simulink model "Controllers_Complete_Comparisons"  (R2021a)
settings: Solver=FixedStepAuto  StartTime=0  StopTime=1  FixedStep=0.002  RelTol=1e-3  EnableMultiTasking=on
PostLoadFcn:
  | qc_set_target_type(getConfigSet(bdroot, 'QUARC Default Target Configuration'));
values from neighbouring files (symbols this model uses):
  L_KF = KalmanFilter(sysest_ct, Q_KF, R_KF)    [LQR_comparison.m]    (also in main.m = Arco_KalmanFilter(sysest_ct, Q_KF, R_KF))
  L_obs = StateObserver(sysest_ct,obs_poles)    [LQR_comparison.m]    (also in main.m = StateObserver_JC(sysest_ct,obs_poles))
  Q_KF = eye(4)*10e-5    [LQR_comparison.m]    (also in main.m = eye(4))
  R_KF = eye(1)*10e-8    [LQR_comparison.m]    (also in main.m = eye(1))
  sysest = load("sysest09c_trick.mat").sysest    [LQR_comparison.m]    (also in main.m)
  sysest_ct = d2c(sysest)    [LQR_comparison.m]    (also in main.m)
  v_a_max = 13    [LQR_comparison.m]    (also in main.m = 15)
undefined symbols (not defined in the file or in its folder): DiscIntNeverNeededParam, HIL, k2, K_lqr, K_lqr_eta, K_lqr_eta_1, K_lqr_eta_2, K_lqr_eta_3, K_lqr_eta_4, K_lqr_x, K_lqr_x_1, K_lqr_x_2, K_lqr_x_3, K_lqr_x_4, K_lqrFF_eta, K_lqrFF_x, K_p, K_pp, K_pp_en_eta, K_pp_en_x, Kr2, L22, qc_get_step_size, sigbuilder_block
libraries: simulink_extras x15, quarc_library x4, cstblocks x1
settings Model: SimulationMode=external  ExtModeTrigDuration=5000  Creator=CFulford  LastModifiedBy=Andrea
settings SolverCC: AlgebraicLoopSolver=TrustRegion  PositivePriorityOrder=on
settings DataIOCC: LimitDataPoints=on  SaveFormat=Array  SignalLoggingSaveFormat=ModelDataLogs  ReturnWorkspaceOutputs=off
settings OptimizationCC: ExpressionDepthLimit=2147483647  InitFltsAndDblsToZero=on  LifeSpan=inf
settings DebuggingCC: SaveWithParameterizedLinksMsg=none  UnderspecifiedInitializationDetection=Classic  MergeDetectMultiDrivingBlocksExec=none  SolverPrmCheckMsg=warning  MultiTaskDSMMsg=warning  MultiTaskCondExecSysMsg=none  FcnCallInpInsideContextMsg=warning  StateNameClashWarn=warning  SFUnexpectedBacktrackingDiag=warning  SFNoUnconditionalDefaultTransitionDiag=warning  SFExecutionAtInitializationDiag=none  SFMachineParentedDataDiag=warning  ArithmeticOperatorsInVariantConditions=warning
settings HardwareCC: ProdBitPerPointer=32  ProdBitPerSizeT=32  ProdBitPerPtrDiffT=32  ProdLargestAtomicFloat=None  ProdIntDivRoundTo=Undefined  ProdEndianess=Unspecified  ProdWordSize=32  ProdHWDeviceType=32-bit Generic
settings ModelReferenceCC: PropagateSignalLabelsOutOfModel=off
settings SFSimCC: SimUseLocalCustomCode=off  CustomCodeUndefinedFunction=UseInterfaceOnly
settings RTWCC: Description=QUARC Win64 Target  SystemTargetFile=quarc_win64.tlc  TemplateMakefile=quarc_default_tmf  RTWUseLocalCustomCode=off
settings CodeAppCC: StateflowObjectComments=on
settings STFCustomTargetCC: TargetPreCompLibLocation=C:\PROGRA~3\QUARC\lib\2019b\win64\release  ConcurrentExecutionCompliant=on  CombineOutputUpdateFcns=on  CPPClassGenCompliant=on  GRTInterface=off  UseToolchainInfoCompliant=off  SystemTargetFile=quarc_win64.tlc
settings GRTTargetCC: TargetPreCompLibLocation=C:\PROGRA~3\QUARC\lib\2019b\win64\release  TargetLangStandard=C89/C90 (ANSI)  ParMdlRefBuildCompliant=off  CompOptLevelCompliant=off  MatFileLogging=off  UseToolchainInfoCompliant=off  ExtMode=on  ExtModeMexFile=quarc_comm
settings ConfigComp: CovMetricSettings=dw  CovSaveCumulativeToWorkspaceVar=on  CovSaveSingleToWorkspaceVar=on  CovExternalEMLEnable=off  CovSFcnEnable=off

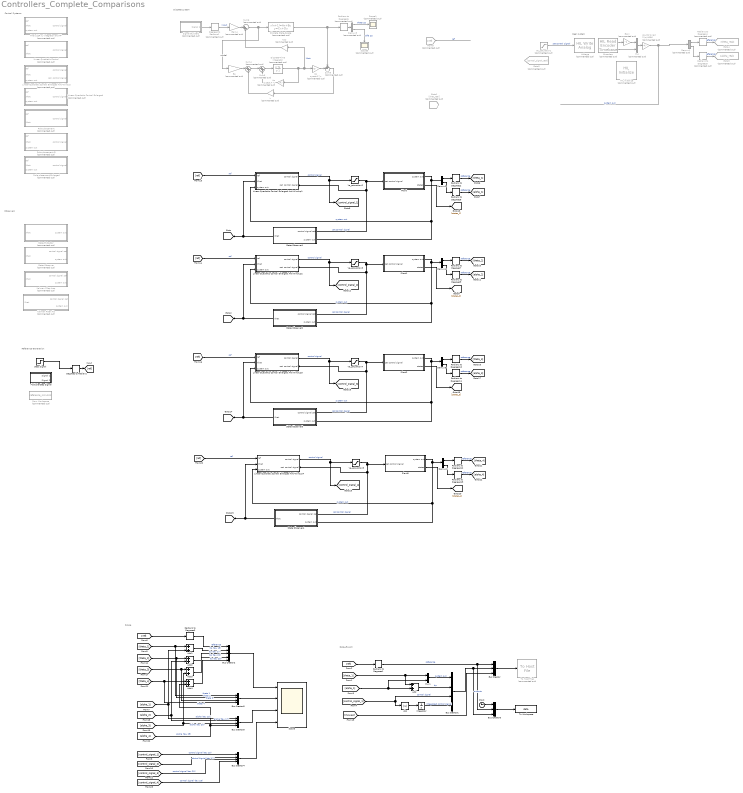
== system Controllers_Complete_Comparisons ==
  note: Real system
  note: Reference Generation
  note: Scope
  note: Control Systems
  note: Observers
  note: Discrete system
  note: model
  note: Data_Export
  Abs : Abs
  Add{,1..4} (5 alike) : Sum
  Ao : Gain  Commented=on  Gain=sysest.A  Multiplication=Matrix(K*u)
  Bo : Gain  Commented=on  Gain=sysest.B  Multiplication=Matrix(K*u)
  Bus Creator : BusCreator  Inputs=3
  Bus Creator{1,3..5} (4 alike) : BusCreator  Inputs=4
  Bus Creator2 : BusCreator  Inputs=5
  Bus Creator6 : BusCreator  Inputs=3
  Clock : Clock
  Co : Gain  Commented=on  Gain=sysest.C  Multiplication=Matrix(K*u)
  Degrees to Radians : simulink_extras/Transformations/Degrees to Radians
  Degrees to Radians1 : simulink_extras/Transformations/Degrees to Radians  Commented=on
  Demux1 : Demux  Commented=on  Outputs=2
  Demux{2,4..6} (4 alike) : Demux  Outputs=2
  Demux3 : Demux  Commented=on  Outputs=2
  Discrete State-Space : DiscreteStateSpace  Commented=on  A=sysest.A  B=sysest.B  C=sysest.C  D=sysest.D  SampleTime=0.002
  Discrete-Time Integrator : DiscreteIntegrator  Commented=on  SampleTime=0.002  ICPrevOutput=DiscIntNeverNeededParam  ICPrevScaledInput=DiscIntNeverNeededParam
  Encoders : quarc_library/Data Acquisition/Generic/Timebases/HIL Read Encoder Timebase  Commented=on  object_name=HIL-1  clock=0  channels=[0:1]  samples_in_buffer=max(ceil(1/qc_get_step_size), 1)  active=on  vector_output=off  data_type_mode=Inherit via back propagation  data_type=double
  Fire's LQR w/ integrator and FF : Subsystem  Commented=on
  From Workspace : FromWorkspace  Commented=on  VariableName=reference_simulink
  From9 : From  Commented=on  GotoTag=ref
  Gain : Gain  Commented=on  Gain=-1
  Gain4 : Gain  Commented=on  Gain=Kr2(1)
  Goto1 : Goto  Commented=on  GotoTag=Xhat_real
  Goto3 : Goto  Commented=on  GotoTag=alpha_real
  Goto4 : Goto  Commented=on  GotoTag=theta_real
  Goto5 : Goto  Commented=on  GotoTag=control_signal_real
  HIL Initialize : quarc_library/Data Acquisition/Generic/Configuration/HIL Initialize  Priority=-99  Commented=on  object_name=HIL-1  board_type=q2_usb  board_number=0  board_options=d0=digital;d1=digital;led=auto;update_rate=normal;decimation=1  exclusive=off  active=off  hardware_clocks=[0]  clock_modes=[]  initial_clock_frequencies=[]  set_clock_params_at_start=off  set_clock_params_at_switch_in=off  set_clock_frequencies_at_start=off  set_clock_frequencies_at_switch_in=off  analog_input_channels=[0:1]  analog_input_configurations=[]  analog_input_maximums=10  analog_input_minimums=-10  set_analog_input_params_at_start=on  set_analog_input_params_at_switch_in=off  analog_output_channels=[0:1]  analog_output_maximums=10  analog_output_minimums=-10  initial_analog_outputs=[0]  final_analog_outputs=[0]  watchdog_analog_outputs=0  set_analog_output_params_at_start=on  set_analog_output_params_at_switch_in=off  set_analog_outputs_at_start=on  set_analog_outputs_at_switch_in=off  set_analog_outputs_at_terminate=on  set_analog_outputs_at_switch_out=off  set_analog_outputs_on_watchdog=off  digital_input_channels=[]  digital_output_channels=[]  digital_output_configuration=[]  initial_digital_outputs=[1]  final_digital_outputs=[1]  watchdog_digital_outputs=[1]  set_digital_output_params_at_start=off  set_digital_output_params_at_switch_in=off  set_digital_outputs_at_start=on  set_digital_outputs_at_switch_in=off  set_digital_outputs_at_terminate=on  set_digital_outputs_at_switch_out=off  set_digital_outputs_on_watchdog=off  encoder_channels=[0:1]  quadrature=[4]  encoder_filter_frequency=[]  initial_encoder_counts=[0]  set_encoder_params_at_start=on  set_encoder_params_at_switch_in=off  set_encoder_counts_at_start=on  set_encoder_counts_at_switch_in=off  pwm_channels=[]  pwm_modes=[0]  pwm_frequency=1/0.020  pwm_configuration=[]  pwm_alignment=[]  pwm_polarity=[]  pwm_leading_deadband=[]  pwm_trailing_deadband=[]  initial_pwm_outputs=[0]  final_pwm_outputs=[0]  watchdog_pwm_outputs=[0]  set_pwm_params_at_start=on  set_pwm_params_at_switch_in=off  set_pwm_outputs_at_start=on  set_pwm_outputs_at_switch_in=off  set_pwm_outputs_at_terminate=on  set_pwm_outputs_at_switch_out=off  set_pwm_outputs_on_watchdog=off  other_output_channels=[]  initial_other_outputs=[]  final_other_outputs=[]  watchdog_other_outputs=[]  set_other_outputs_at_start=off  set_other_outputs_at_switch_in=off  set_other_outputs_at_terminate=off  set_other_outputs_at_switch_out=off  set_other_outputs_on_watchdog=off
  Integrator : Integrator
  Kalman Filter Alp : Subsystem  Commented=on
  Kalman Filter Arco : Subsystem  Commented=on
  Kpp : Gain  Commented=on  Gain=k2  Multiplication=Matrix(K*u)
  L : Gain  Commented=on  Gain=L22  Multiplication=Matrix(K*u)
  Linear Quadratic Control : Subsystem  Commented=on
  Linear Quadratic Control Enlarged : Subsystem  Commented=on
  Linear Quadratic Control Enlarged Anti-Windup : Subsystem  Commented=on
      settings: PortSchema="{\"entries\":[{\"content\":{\"sides\":[{\"content\":{\"connectorIds\":[\"In1\",\"In2\",\"In3\"]},\"type\":\"ConnectorPlacement.EquallySpacedRectSide\",\"uuid\":\"15b51522-458a-4f7c-a290-9c80724aecba\"},{\"content\":{\"connectorIds\":[\"Out1\",\"In4\"],\"side\":\"RIGHT\"},\"type\":\"ConnectorPlacement.EquallySpacedRectSide\",\"uuid\":\"ee497df3-c1d4-4daa-9165-c0ca341e658c\"},{\"content\":{\"connectorIds\":[],\"side\":\"TOP\"},\"type\":\"ConnectorPlacement.EquallySpacedRectSide\",\"uuid\":\"946f2086-2c09-46d1-b933-0f6497ae0c76\"}]},\"type\":\"ConnectorPlacement.EquallySpacedConnector\",\"uuid\":\"4633a66e-f116-47af-8162-46d62cad4c11\"}],\"packageUris\":[\"http://schema.mathworks.com/mf0/Connector/R2020b\"],\"version\":\"1.0\"}"
  Linear Quadratic Control Enlarged Anti-Windup1 : Subsystem
      settings: PortSchema="{\"entries\":[{\"content\":{\"sides\":[{\"content\":{\"connectorIds\":[\"In1\",\"In2\",\"In3\"]},\"type\":\"ConnectorPlacement.EquallySpacedRectSide\",\"uuid\":\"15b51522-458a-4f7c-a290-9c80724aecba\"},{\"content\":{\"connectorIds\":[\"Out1\",\"In4\"],\"side\":\"RIGHT\"},\"type\":\"ConnectorPlacement.EquallySpacedRectSide\",\"uuid\":\"ee497df3-c1d4-4daa-9165-c0ca341e658c\"},{\"content\":{\"connectorIds\":[],\"side\":\"TOP\"},\"type\":\"ConnectorPlacement.EquallySpacedRectSide\",\"uuid\":\"946f2086-2c09-46d1-b933-0f6497ae0c76\"}]},\"type\":\"ConnectorPlacement.EquallySpacedConnector\",\"uuid\":\"4633a66e-f116-47af-8162-46d62cad4c11\"}],\"packageUris\":[\"http://schema.mathworks.com/mf0/Connector/R2020b\"],\"version\":\"1.0\"}"
  Linear Quadratic Control Enlarged Anti-Windup2 : Subsystem
      settings: PortSchema="{\"entries\":[{\"content\":{\"sides\":[{\"content\":{\"connectorIds\":[\"In1\",\"In2\",\"In3\"]},\"type\":\"ConnectorPlacement.EquallySpacedRectSide\",\"uuid\":\"15b51522-458a-4f7c-a290-9c80724aecba\"},{\"content\":{\"connectorIds\":[\"Out1\",\"In4\"],\"side\":\"RIGHT\"},\"type\":\"ConnectorPlacement.EquallySpacedRectSide\",\"uuid\":\"ee497df3-c1d4-4daa-9165-c0ca341e658c\"},{\"content\":{\"connectorIds\":[],\"side\":\"TOP\"},\"type\":\"ConnectorPlacement.EquallySpacedRectSide\",\"uuid\":\"946f2086-2c09-46d1-b933-0f6497ae0c76\"}]},\"type\":\"ConnectorPlacement.EquallySpacedConnector\",\"uuid\":\"4633a66e-f116-47af-8162-46d62cad4c11\"}],\"packageUris\":[\"http://schema.mathworks.com/mf0/Connector/R2020b\"],\"version\":\"1.0\"}"
  Linear Quadratic Control Enlarged Anti-Windup3 : Subsystem
      settings: PortSchema="{\"entries\":[{\"content\":{\"sides\":[{\"content\":{\"connectorIds\":[\"In1\",\"In2\",\"In3\"]},\"type\":\"ConnectorPlacement.EquallySpacedRectSide\",\"uuid\":\"15b51522-458a-4f7c-a290-9c80724aecba\"},{\"content\":{\"connectorIds\":[\"Out1\",\"In4\"],\"side\":\"RIGHT\"},\"type\":\"ConnectorPlacement.EquallySpacedRectSide\",\"uuid\":\"ee497df3-c1d4-4daa-9165-c0ca341e658c\"},{\"content\":{\"connectorIds\":[],\"side\":\"TOP\"},\"type\":\"ConnectorPlacement.EquallySpacedRectSide\",\"uuid\":\"946f2086-2c09-46d1-b933-0f6497ae0c76\"}]},\"type\":\"ConnectorPlacement.EquallySpacedConnector\",\"uuid\":\"4633a66e-f116-47af-8162-46d62cad4c11\"}],\"packageUris\":[\"http://schema.mathworks.com/mf0/Connector/R2020b\"],\"version\":\"1.0\"}"
  Linear Quadratic Control Enlarged Anti-Windup4 : Subsystem
      settings: PortSchema="{\"entries\":[{\"content\":{\"sides\":[{\"content\":{\"connectorIds\":[\"In1\",\"In2\",\"In3\"]},\"type\":\"ConnectorPlacement.EquallySpacedRectSide\",\"uuid\":\"15b51522-458a-4f7c-a290-9c80724aecba\"},{\"content\":{\"connectorIds\":[\"Out1\",\"In4\"],\"side\":\"RIGHT\"},\"type\":\"ConnectorPlacement.EquallySpacedRectSide\",\"uuid\":\"ee497df3-c1d4-4daa-9165-c0ca341e658c\"},{\"content\":{\"connectorIds\":[],\"side\":\"TOP\"},\"type\":\"ConnectorPlacement.EquallySpacedRectSide\",\"uuid\":\"946f2086-2c09-46d1-b933-0f6497ae0c76\"}]},\"type\":\"ConnectorPlacement.EquallySpacedConnector\",\"uuid\":\"4633a66e-f116-47af-8162-46d62cad4c11\"}],\"packageUris\":[\"http://schema.mathworks.com/mf0/Connector/R2020b\"],\"version\":\"1.0\"}"
  Multiple-Step Signal : Subsystem  Tag=STV Subsys  LoadFcn=sigbuilder_block('load');  StartFcn=sigbuilder_block('start');  StopFcn=sigbuilder_block('stop');  ClipboardFcn=sigbuilder_block('clipboard');  mask(Sigbuilder block){tuvar=[0:10]}
      mask help: Simulink:masks:SigbuilderBlock_MD
      mask init:
      | if ~strcmp(get_param(bdroot(gcbh),'SimulationStatus'),'stopped') tuvar = sigbuilder_block('maskInit'); end
      settings: CopyFcn=sigbuilder_block('copy');  DeleteFcn=sigbuilder_block('delete');  ModelCloseFcn=sigbuilder_block('modelClose');  PreSaveFcn=sigbuilder_block('preSave');  PauseFcn=sigbuilder_block('pause');  ContinueFcn=sigbuilder_block('continue');  NameChangeFcn=sigbuilder_block('namechange');  OpenFcn=sigbuilder_block('open',[6 30 1428 681.75 ]);  CloseFcn=sigbuilder_block('close');
      mask Display: plot(0, 0, 100, 100,[2, 2, 32, 32, 2], [68, 8, 8, 68, 68],[32, 2], [38, 38], [32, 19, 2],[53, 60, 44], [32, 17, 17, 2],[16, 16, 31, 31]);txt = getActiveGroup(gcbh);text(2, 100, txt,'verticalAlignment', 'top');
  Mux : Mux  Commented=on  Inputs=2
  Mux1 : Mux  Inputs=2
  Plant : Subsystem
  Plant1 : Subsystem
  Plant2 : Subsystem
  Plant3 : Subsystem
  Pole placement : Subsystem  Commented=on
  Pole placement Enlarged : Subsystem  Commented=on
  Pole placement PI : Subsystem  Commented=on
  Radians to Degrees{1..3,7..13} (10 alike) : simulink_extras/Transformations/Radians to Degrees
  Radians to Degrees4 : simulink_extras/Transformations/Radians to Degrees  Commented=on
  Radians to Degrees5 : simulink_extras/Transformations/Radians to Degrees  Commented=on
  Radians to Degrees6 : simulink_extras/Transformations/Radians to Degrees  Commented=on
  Scope : Scope  NumInputPorts=4
  Scope1 : Scope  Commented=on
  Scope3 : Scope  Commented=on
  Signal Builder1 : Subsystem  Tag=STV Subsys  Commented=on  LoadFcn=sigbuilder_block('load');  StartFcn=sigbuilder_block('start');  StopFcn=sigbuilder_block('stop');  ClipboardFcn=sigbuilder_block('clipboard');  mask(Sigbuilder block){tuvar=[0:10]}
      mask help: Simulink:masks:SigbuilderBlock_MD
      mask init:
      | if ~strcmp(get_param(bdroot(gcbh),'SimulationStatus'),'stopped') tuvar = sigbuilder_block('maskInit'); end
      settings: CopyFcn=sigbuilder_block('copy');  DeleteFcn=sigbuilder_block('delete');  ModelCloseFcn=sigbuilder_block('modelClose');  PreSaveFcn=sigbuilder_block('preSave');  PauseFcn=sigbuilder_block('pause');  ContinueFcn=sigbuilder_block('continue');  NameChangeFcn=sigbuilder_block('namechange');  OpenFcn=sigbuilder_block('open',[437.6 199.2 550.4 400 ]);  CloseFcn=sigbuilder_block('close');
      mask Display: plot(0, 0, 100, 100,[2, 2, 32, 32, 2], [68, 8, 8, 68, 68],[32, 2], [38, 38], [32, 19, 2],[53, 60, 44], [32, 17, 17, 2],[16, 16, 31, 31]);txt = getActiveGroup(gcbh);text(2, 100, txt,'verticalAlignment', 'top');
  State Extractor : Subsystem  Commented=on
  State Observer : Subsystem  Commented=on
  State Observer1 : Subsystem
  State Observer2 : Subsystem
  State Observer3 : Subsystem
  State Observer4 : Subsystem
  Step Signal : Step  Time=0.2  After=45  SampleTime=0
  Sum3 : Sum  Commented=on  Inputs=|++
  Sum4 : Sum  Commented=on  Inputs=|++
  Sum5 : Sum  Commented=on  Inputs=+-|
  Sum6 : Sum  Commented=on  Inputs=|+-
  To Host File1 : quarc_library/Sinks/To Host/To Host File  Commented=on  file_name=Sine tests\Sine_24_in_theta_alpha.mat  variable_name=data  decimation=1  sample_time=-1  file_format=MAT-file v.4  options=No header or footer  append=off  final_file_name=Sine tests\Sine_24_in_theta_alpha.mat  bitrate=2000000
  To Workspace : ToWorkspace  VariableName=data  SampleTime=-1
  Va_saturation1 : Saturate  Commented=on  UpperLimit=v_a_max  LowerLimit=-v_a_max
  Va_saturation{2..5} (4 alike) : Saturate  UpperLimit=v_a_max  LowerLimit=-v_a_max
  Voltage : quarc_library/Data Acquisition/Generic/Immediate I//O/HIL Write Analog  Commented=on  object_name=HIL-1  channels=0  sample_time=-1  active=off  vector_input=off
  counts to rad : Gain  Commented=on  Gain=2*pi/4096
  wires:
  Bus Creator2/1 -> Scope/1
  Bus Creator3/1 -> Scope/3
  ? -> Goto5/1, Va_saturation1/1  "control signal"
  Demux2/1 -> Radians to Degrees2/1
  Linear Quadratic Control Enlarged Anti-Windup1/1(" control signal") -> [control_signal_1], Va_saturation2/1  "control signal"
  [ref] -> Linear Quadratic Control Enlarged Anti-Windup1/1(ref)  "ref"
  [control_signal_2] -> Bus Creator4/2  "control signal (tau 17)"
  [alpha_2] -> Add2/2, Bus Creator3/2  "alpha (tau 17)"
  Demux1/1 -> Radians to Degrees4/1
  counts to rad/1 -> Demux1/1  "system out"
  [theta_2] -> Bus Creator5/2, Add2/1  "theta 2"
  Va_saturation2/1 -> Linear Quadratic Control Enlarged Anti-Windup1/4(sat  control signal), State Observer1/1(control signal sat), Plant/1(sat control signal)  "sat control signal"
  Demux1/2 -> Radians to Degrees5/1
  Plant/1(system out) -> Linear Quadratic Control Enlarged Anti-Windup1/3(system out), State Observer1/2(system out), Demux2/1  "system out"
  [control_signal_1] -> Bus Creator4/1  "control signal (tau 15)"
  Degrees to Radians/1 -> [ref]
  Bus Creator4/1 -> Scope/4
  Radians to Degrees3/1 -> Bus Creator2/1  "reference"
  Va_saturation1/1 -> Voltage/1  "sat control signal"
  [alpha_1] -> Bus Creator3/1, Add1/2  "alpha (tau 15)"
  [theta_1] -> Bus Creator5/1, Add1/1  "theta 1"
  Demux2/2 -> Radians to Degrees8/1
  Sum5/1 -> L/1
  Demux3/1 -> Scope1/1  "theta pp"
  Sum6/1 -> Discrete State-Space/1, Bo/1
  L/1 -> Sum4/2
  Discrete State-Space/1 -> Radians to Degrees6/1, Sum5/1
  Sum4/1 -> Sum3/1
  Sum3/1 -> Discrete-Time Integrator/1
  Degrees to Radians1/1 -> Gain4/1  "input"
  Co/1 -> Sum5/2
  Demux3/2 -> Scope3/1  "alfa pp"
  Signal Builder1/1(Signal 1) -> Degrees to Radians1/1
  Kpp/1 -> Sum6/2
  Bo/1 -> Sum4/1
  Discrete-Time Integrator/1 -> Ao/1, Kpp/1, Co/1  "Xhat"
  Gain4/1 -> Sum6/1
  Ao/1 -> Sum3/2
  Radians to Degrees6/1 -> Demux3/1
  From9/1 -> ?  "ref"
  Step Signal/1 -> Degrees to Radians/1
  Add1/1 -> Bus Creator2/2  "tip (tau 15)"
  Add2/1 -> Bus Creator2/3  "tip (tau 17)"
  [ref] -> Radians to Degrees3/1
  Radians to Degrees2/1 -> [theta_1]  "reference"
  Radians to Degrees8/1 -> [alpha_1]  "reference"
  ? -> Goto1/1
  Bus Creator/1 -> To Host File1/1
  [theta_1] -> Add/1, Mux1/1
  [ref] -> Radians to Degrees1/1
  Abs/1 -> Integrator/1
  [control_signal_1] -> Abs/1, Bus Creator1/3  "control signal"
  Mux1/1 -> Bus Creator1/1  "system out"
  Integrator/1 -> Bus Creator1/4  "integrated control signal"
  Radians to Degrees1/1 -> Bus Creator/1, Bus Creator6/2  "reference"
  Bus Creator1/1 -> Bus Creator/2, Bus Creator6/3  "outputs"
  [Xhat_real] -> Bus Creator/3
  Add/1 -> Bus Creator1/2  "tip"
  [alpha_1] -> Add/2, Mux1/2
  Gain/1 -> Mux/1
  Mux/1 -> counts to rad/1
  Encoders/2 -> Mux/2
  Encoders/1 -> Gain/1
  Radians to Degrees4/1 -> Goto4/1  "reference"
  Radians to Degrees5/1 -> Goto3/1  "reference"
  State Observer1/1(Xhat) -> Linear Quadratic Control Enlarged Anti-Windup1/2(Xhat), [Xhat_1]
  Bus Creator5/1 -> Scope/2
  Plant/2(states) -> [states_1]
  Radians to Degrees7/1 -> [theta_2]  "reference"
  Demux4/2 -> Radians to Degrees9/1
  Va_saturation3/1 -> Linear Quadratic Control Enlarged Anti-Windup2/4(sat  control signal), State Observer2/1(control signal sat), Plant1/1(sat control signal)  "sat control signal"
  Demux4/1 -> Radians to Degrees7/1
  [ref] -> Linear Quadratic Control Enlarged Anti-Windup2/1(ref)  "ref"
  Linear Quadratic Control Enlarged Anti-Windup2/1(" control signal") -> [control_signal_2], Va_saturation3/1  "control signal"
  Plant1/1(system out) -> Linear Quadratic Control Enlarged Anti-Windup2/3(system out), State Observer2/2(system out), Demux4/1  "system out"
  State Observer2/1(Xhat) -> Linear Quadratic Control Enlarged Anti-Windup2/2(Xhat), [Xhat_2]
  Plant1/2(states) -> [states_2]
  Radians to Degrees9/1 -> [alpha_2]  "reference"
  Radians to Degrees10/1 -> [theta_3]  "reference"
  Demux5/2 -> Radians to Degrees11/1
  Va_saturation4/1 -> Linear Quadratic Control Enlarged Anti-Windup3/4(sat  control signal), State Observer3/1(control signal sat), Plant2/1(sat control signal)  "sat control signal"
  Demux5/1 -> Radians to Degrees10/1
  [ref] -> Linear Quadratic Control Enlarged Anti-Windup3/1(ref)  "ref"
  Linear Quadratic Control Enlarged Anti-Windup3/1(" control signal") -> [control_signal_3], Va_saturation4/1  "control signal"
  Plant2/1(system out) -> Linear Quadratic Control Enlarged Anti-Windup3/3(system out), State Observer3/2(system out), Demux5/1  "system out"
  State Observer3/1(Xhat) -> Linear Quadratic Control Enlarged Anti-Windup3/2(Xhat), [Xhat_3]
  Plant2/2(states) -> [states_3]
  Radians to Degrees11/1 -> [alpha_3]  "reference"
  [theta_3] -> Bus Creator5/3, Add3/1  "theta 3"
  Add3/1 -> Bus Creator2/4  "tip (tau 20)"
  [alpha_3] -> Add3/2, Bus Creator3/3  "alpha (tau 20)"
  [control_signal_3] -> Bus Creator4/3  "control signal (tau 20)"
  Bus Creator6/1 -> To Workspace/1
  Clock/1 -> Bus Creator6/1
  Linear Quadratic Control Enlarged Anti-Windup4/1(" control signal") -> [control_signal_4], Va_saturation5/1  "control signal"
  Plant3/2(states) -> [states_4]
  Radians to Degrees13/1 -> [alpha_4]  "reference"
  State Observer4/1(Xhat) -> Linear Quadratic Control Enlarged Anti-Windup4/2(Xhat), [Xhat_4]
  Demux6/1 -> Radians to Degrees12/1
  Va_saturation5/1 -> Linear Quadratic Control Enlarged Anti-Windup4/4(sat  control signal), State Observer4/1(control signal sat), Plant3/1(sat control signal)  "sat control signal"
  Demux6/2 -> Radians to Degrees13/1
  Radians to Degrees12/1 -> [theta_4]  "reference"
  Plant3/1(system out) -> Linear Quadratic Control Enlarged Anti-Windup4/3(system out), State Observer4/2(system out), Demux6/1  "system out"
  [ref] -> Linear Quadratic Control Enlarged Anti-Windup4/1(ref)  "ref"
  [theta_4] -> Bus Creator5/4, Add4/1  "theta 4"
  Add4/1 -> Bus Creator2/5  "tip (tau 25)"
  [alpha_4] -> Add4/2, Bus Creator3/4  "alpha (tau 25)"
  [control_signal_4] -> Bus Creator4/4  "control signal (tau 25)"

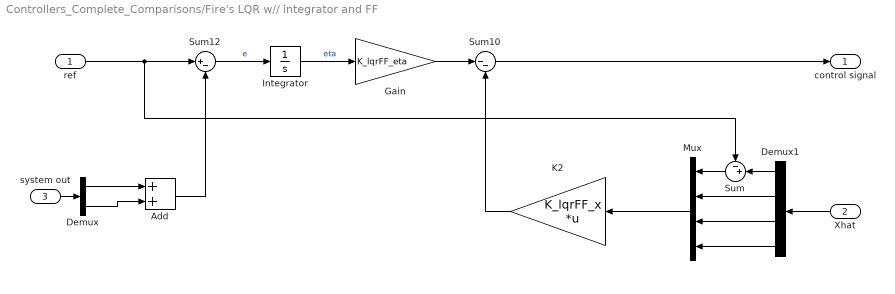
== system Controllers_Complete_Comparisons/Fire's LQR w// integrator and FF ==
  ref : Inport
  Xhat : Inport  Port=2
  system out : Inport  Port=3
  Add : Sum
  Demux : Demux  Outputs=2
  Demux1 : Demux
  Gain : Gain  Gain=K_lqrFF_eta
  Integrator : Integrator
  K2 : Gain  Gain=K_lqrFF_x  Multiplication=Matrix(K*u)
  Mux : Mux
  Sum : Sum  Inputs=-+|
  Sum10 : Sum  Inputs=|--
  Sum12 : Sum  Inputs=|+-
  " control signal" : Outport
  wires:
  ref/1 -> Sum/1, Sum12/1
  Gain/1 -> Sum10/1
  Integrator/1 -> Gain/1  "eta"
  Sum10/1 -> " control signal"/1
  K2/1 -> Sum10/2
  Add/1 -> Sum12/2
  Sum12/1 -> Integrator/1  "e"
  Xhat/1 -> Demux1/1
  system out/1 -> Demux/1
  Demux/2 -> Add/2
  Demux/1 -> Add/1
  Mux/1 -> K2/1
  Demux1/1 -> Sum/2
  Sum/1 -> Mux/1
  Demux1/2 -> Mux/2
  Demux1/4 -> Mux/4
  Demux1/3 -> Mux/3

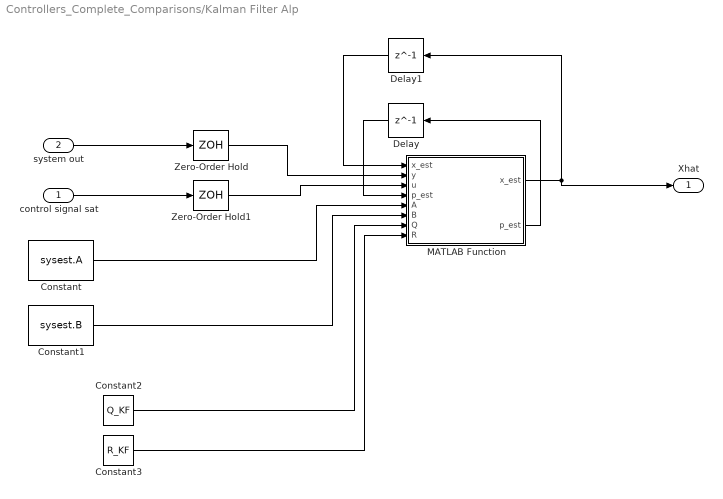
== system Controllers_Complete_Comparisons/Kalman Filter Alp ==
  control signal sat : Inport
  system out : Inport  Port=2
  Constant : Constant  Value=sysest.A
  Constant1 : Constant  Value=sysest.B
  Constant2 : Constant  Value=Q_KF
  Constant3 : Constant  Value=R_KF
  Delay : Delay  DelayLength=1  InitialCondition=eye(4)
  Delay1 : Delay  DelayLength=1  InitialCondition=[0;0;0;0]
  MATLAB Function : MATLAB Function  TreatAsAtomicUnit=on
  Zero-Order Hold : ZeroOrderHold  SampleTime=0.002
  Zero-Order Hold1 : ZeroOrderHold  SampleTime=0.002
  Xhat : Outport
  wires:
  MATLAB Function/1(x_est) -> Xhat/1, Delay1/1
  Delay/1 -> MATLAB Function/4("p_est ")
  MATLAB Function/2(p_est) -> Delay/1
  Zero-Order Hold1/1 -> MATLAB Function/3(u)
  Constant1/1 -> MATLAB Function/6(B)
  Delay1/1 -> MATLAB Function/1("x_est ")
  Constant/1 -> MATLAB Function/5(A)
  Zero-Order Hold/1 -> MATLAB Function/2(y)
  control signal sat/1 -> Zero-Order Hold1/1
  system out/1 -> Zero-Order Hold/1
  Constant2/1 -> MATLAB Function/7(Q)
  Constant3/1 -> MATLAB Function/8(R)

== system Controllers_Complete_Comparisons/Kalman Filter Arco ==
  control signal sat : Inport  PortDimensions=1
  system out : Inport  Port=2  PortDimensions=2
  Add : Sum  Inputs=+++
  Gain : Gain  Gain=sysest_ct.B  Multiplication=Matrix(K*u) (u vector)
  Gain1 : Gain  Gain=L_KF  Multiplication=Matrix(K*u) (u vector)
  Gain2 : Gain  Gain=sysest_ct.A - L_KF * sysest_ct.C  Multiplication=Matrix(K*u) (u vector)
  Integrator : Integrator
  Xhat : Outport  PortDimensions=4
  wires:
  Gain2/1 -> Add/1
  Integrator/1 -> Gain2/1, Xhat/1  "x_hat"
  Add/1 -> Integrator/1  "x_hat_dot"
  Gain/1 -> Add/2
  control signal sat/1 -> Gain/1
  Gain1/1 -> Add/3
  system out/1 -> Gain1/1

== system Controllers_Complete_Comparisons/Linear Quadratic Control ==
  ref : Inport
  Xhat : Inport  Port=2
  Demux : Demux
  Gain3 : Gain  Gain=-K_lqr  Multiplication=Matrix(K*u)
  Mux : Mux
  Sum1 : Sum  Inputs=-+|
  " control signal" : Outport
  wires:
  ref/1 -> Sum1/1
  Xhat/1 -> Demux/1
  Demux/1 -> Sum1/2  "theta"
  Demux/2 -> Mux/2  "theta_dot"
  Demux/3 -> Mux/3  "alpha"
  Demux/4 -> Mux/4  "alpha_dot"
  Gain3/1 -> " control signal"/1
  Sum1/1 -> Mux/1
  Mux/1 -> Gain3/1

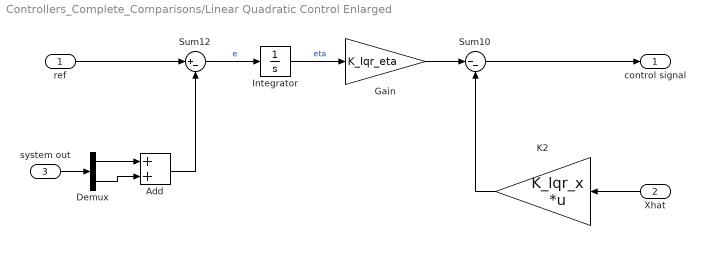
== system Controllers_Complete_Comparisons/Linear Quadratic Control Enlarged ==
  ref : Inport
  Xhat : Inport  Port=2
  system out : Inport  Port=3
  Add : Sum
  Demux : Demux  Outputs=2
  Gain : Gain  Gain=K_lqr_eta
  Integrator : Integrator
  K2 : Gain  Gain=K_lqr_x  Multiplication=Matrix(K*u)
  Sum10 : Sum  Inputs=|--
  Sum12 : Sum  Inputs=|+-
  " control signal" : Outport
  wires:
  ref/1 -> Sum12/1
  Gain/1 -> Sum10/1
  Integrator/1 -> Gain/1  "eta"
  Sum10/1 -> " control signal"/1
  K2/1 -> Sum10/2
  Add/1 -> Sum12/2
  Sum12/1 -> Integrator/1  "e"
  Xhat/1 -> K2/1
  system out/1 -> Demux/1
  Demux/2 -> Add/2
  Demux/1 -> Add/1

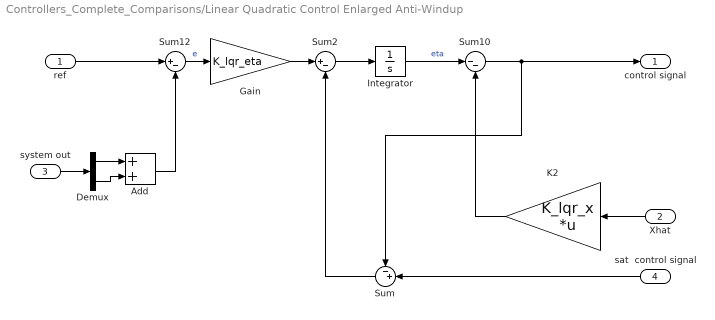
== system Controllers_Complete_Comparisons/Linear Quadratic Control Enlarged Anti-Windup ==
  ref : Inport
  Xhat : Inport  Port=2
  system out : Inport  Port=3
  sat  control signal : Inport  Port=4
  Add : Sum
  Demux : Demux  Outputs=2
  Gain : Gain  Gain=K_lqr_eta
  Integrator : Integrator
  K2 : Gain  Gain=K_lqr_x  Multiplication=Matrix(K*u)
  Sum : Sum  Inputs=-+|
  Sum10 : Sum  Inputs=|--
  Sum12 : Sum  Inputs=|+-
  Sum2 : Sum  Inputs=|+-
  " control signal" : Outport
  wires:
  ref/1 -> Sum12/1
  Integrator/1 -> Sum10/1  "eta"
  K2/1 -> Sum10/2
  Add/1 -> Sum12/2
  Xhat/1 -> K2/1
  system out/1 -> Demux/1
  Demux/2 -> Add/2
  Demux/1 -> Add/1
  sat  control signal/1 -> Sum/2
  Sum10/1 -> Sum/1, " control signal"/1
  Sum12/1 -> Gain/1  "e"
  Sum2/1 -> Integrator/1
  Sum/1 -> Sum2/2
  Gain/1 -> Sum2/1

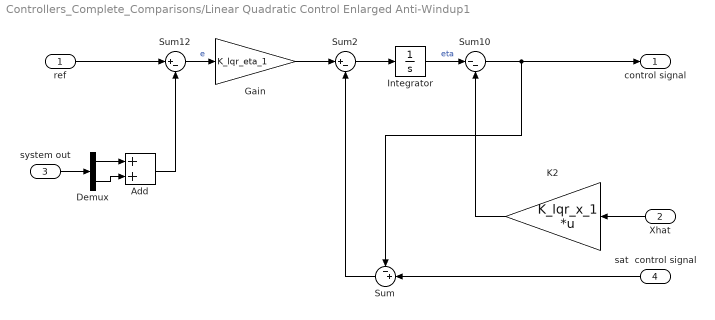
== system Controllers_Complete_Comparisons/Linear Quadratic Control Enlarged Anti-Windup1 ==
  ref : Inport
  Xhat : Inport  Port=2
  system out : Inport  Port=3
  sat  control signal : Inport  Port=4
  Add : Sum
  Demux : Demux  Outputs=2
  Gain : Gain  Gain=K_lqr_eta_1
  Integrator : Integrator
  K2 : Gain  Gain=K_lqr_x_1  Multiplication=Matrix(K*u)
  Sum : Sum  Inputs=-+|
  Sum10 : Sum  Inputs=|--
  Sum12 : Sum  Inputs=|+-
  Sum2 : Sum  Inputs=|+-
  " control signal" : Outport
  wires:
  ref/1 -> Sum12/1
  Integrator/1 -> Sum10/1  "eta"
  K2/1 -> Sum10/2
  Add/1 -> Sum12/2
  Xhat/1 -> K2/1
  system out/1 -> Demux/1
  Demux/2 -> Add/2
  Demux/1 -> Add/1
  sat  control signal/1 -> Sum/2
  Sum10/1 -> Sum/1, " control signal"/1
  Sum12/1 -> Gain/1  "e"
  Sum2/1 -> Integrator/1
  Sum/1 -> Sum2/2
  Gain/1 -> Sum2/1

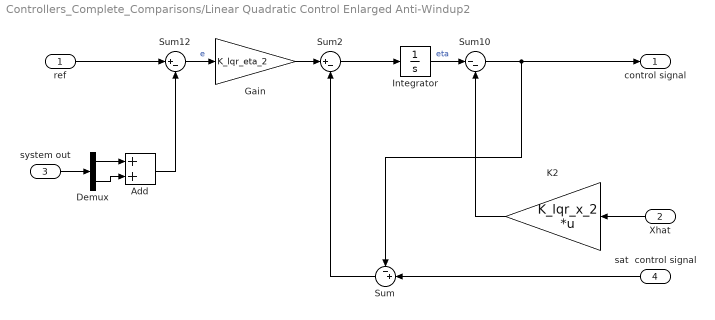
== system Controllers_Complete_Comparisons/Linear Quadratic Control Enlarged Anti-Windup2 ==
  ref : Inport
  Xhat : Inport  Port=2
  system out : Inport  Port=3
  sat  control signal : Inport  Port=4
  Add : Sum
  Demux : Demux  Outputs=2
  Gain : Gain  Gain=K_lqr_eta_2
  Integrator : Integrator
  K2 : Gain  Gain=K_lqr_x_2  Multiplication=Matrix(K*u)
  Sum : Sum  Inputs=-+|
  Sum10 : Sum  Inputs=|--
  Sum12 : Sum  Inputs=|+-
  Sum2 : Sum  Inputs=|+-
  " control signal" : Outport
  wires:
  ref/1 -> Sum12/1
  Integrator/1 -> Sum10/1  "eta"
  K2/1 -> Sum10/2
  Add/1 -> Sum12/2
  Xhat/1 -> K2/1
  system out/1 -> Demux/1
  Demux/2 -> Add/2
  Demux/1 -> Add/1
  sat  control signal/1 -> Sum/2
  Sum10/1 -> Sum/1, " control signal"/1
  Sum12/1 -> Gain/1  "e"
  Sum2/1 -> Integrator/1
  Sum/1 -> Sum2/2
  Gain/1 -> Sum2/1

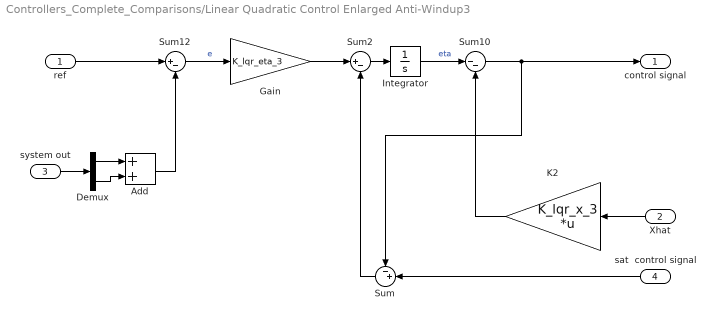
== system Controllers_Complete_Comparisons/Linear Quadratic Control Enlarged Anti-Windup3 ==
  ref : Inport
  Xhat : Inport  Port=2
  system out : Inport  Port=3
  sat  control signal : Inport  Port=4
  Add : Sum
  Demux : Demux  Outputs=2
  Gain : Gain  Gain=K_lqr_eta_3
  Integrator : Integrator
  K2 : Gain  Gain=K_lqr_x_3  Multiplication=Matrix(K*u)
  Sum : Sum  Inputs=-+|
  Sum10 : Sum  Inputs=|--
  Sum12 : Sum  Inputs=|+-
  Sum2 : Sum  Inputs=|+-
  " control signal" : Outport
  wires:
  ref/1 -> Sum12/1
  Integrator/1 -> Sum10/1  "eta"
  K2/1 -> Sum10/2
  Add/1 -> Sum12/2
  Xhat/1 -> K2/1
  system out/1 -> Demux/1
  Demux/2 -> Add/2
  Demux/1 -> Add/1
  sat  control signal/1 -> Sum/2
  Sum10/1 -> Sum/1, " control signal"/1
  Sum12/1 -> Gain/1  "e"
  Sum2/1 -> Integrator/1
  Sum/1 -> Sum2/2
  Gain/1 -> Sum2/1

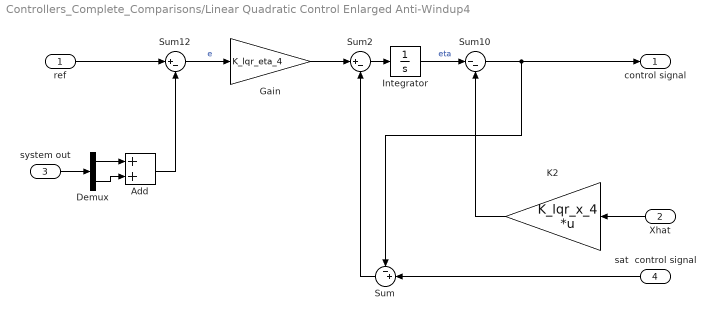
== system Controllers_Complete_Comparisons/Linear Quadratic Control Enlarged Anti-Windup4 ==
  ref : Inport
  Xhat : Inport  Port=2
  system out : Inport  Port=3
  sat  control signal : Inport  Port=4
  Add : Sum
  Demux : Demux  Outputs=2
  Gain : Gain  Gain=K_lqr_eta_4
  Integrator : Integrator
  K2 : Gain  Gain=K_lqr_x_4  Multiplication=Matrix(K*u)
  Sum : Sum  Inputs=-+|
  Sum10 : Sum  Inputs=|--
  Sum12 : Sum  Inputs=|+-
  Sum2 : Sum  Inputs=|+-
  " control signal" : Outport
  wires:
  ref/1 -> Sum12/1
  Integrator/1 -> Sum10/1  "eta"
  K2/1 -> Sum10/2
  Add/1 -> Sum12/2
  Xhat/1 -> K2/1
  system out/1 -> Demux/1
  Demux/2 -> Add/2
  Demux/1 -> Add/1
  sat  control signal/1 -> Sum/2
  Sum10/1 -> Sum/1, " control signal"/1
  Sum12/1 -> Gain/1  "e"
  Sum2/1 -> Integrator/1
  Sum/1 -> Sum2/2
  Gain/1 -> Sum2/1

== system Controllers_Complete_Comparisons/Multiple-Step Signal ==
  Demux : Demux  Tag=STV Demux  Outputs=2
      settings: DisplayOption=none
  FromWs : FromWorkspace  Tag=STV FromWs  VariableName=tuvar
      SigBuilderData=|
      | common.afterFinalStr = 'Extrapolate'
      | common.sampleTime = 0
      | dataSet.timeRange = [0 10]
      | dataSet.name = 'Group 1'
      | sbobj.Groups.Name = 'Group 1'
      | sbobj.Groups.Signals(1).Name = 'Signal 1'
      | sbobj.Groups.Signals(1).XData = [0 1 1 3 3 7 7 8.5 8.5 10]
      | sbobj.Groups.Signals(1).YData = [0.005 0.005 40 40 -30 -30 0 0 23 23]
      | sbobj.Groups.Signals(2).Name = 'Signal 2'
      | sbobj.Groups.Signals(2).XData = [0 1 1 1.52 10]
      | sbobj.Groups.Signals(2).YData = [0 0 -40 -40 -40]
  Signal 1 : Outport  Tag=STV Outport
  Signal 2 : Outport  Tag=STV Outport  Port=2
  wires:
  Demux/1 -> Signal 1/1
  FromWs/1 -> Demux/1
  Demux/2 -> Signal 2/1

== system Controllers_Complete_Comparisons/Plant ==
  sat control signal : Inport
  A1 : Gain  Gain=sysest_ct.A  Multiplication=Matrix(K*u)
  B1 : Gain  Gain=sysest_ct.B  Multiplication=Matrix(K*u)
  C1 : Gain  Gain=sysest_ct.C  Multiplication=Matrix(K*u)
  Integrator2 : Integrator
  Sum7 : Sum  Inputs=|++
  system out : Outport
  states : Outport  Port=2
  wires:
  Sum7/1 -> Integrator2/1
  B1/1 -> Sum7/1
  Integrator2/1 -> states/1, A1/1, C1/1  "xhat"
  C1/1 -> system out/1  "y"
  A1/1 -> Sum7/2
  sat control signal/1 -> B1/1

== system Controllers_Complete_Comparisons/Plant1 ==
  sat control signal : Inport
  A1 : Gain  Gain=sysest_ct.A  Multiplication=Matrix(K*u)
  B1 : Gain  Gain=sysest_ct.B  Multiplication=Matrix(K*u)
  C1 : Gain  Gain=sysest_ct.C  Multiplication=Matrix(K*u)
  Integrator2 : Integrator
  Sum7 : Sum  Inputs=|++
  system out : Outport
  states : Outport  Port=2
  wires:
  Sum7/1 -> Integrator2/1
  B1/1 -> Sum7/1
  Integrator2/1 -> states/1, A1/1, C1/1  "xhat"
  C1/1 -> system out/1  "y"
  A1/1 -> Sum7/2
  sat control signal/1 -> B1/1

== system Controllers_Complete_Comparisons/Plant2 ==
  sat control signal : Inport
  A1 : Gain  Gain=sysest_ct.A  Multiplication=Matrix(K*u)
  B1 : Gain  Gain=sysest_ct.B  Multiplication=Matrix(K*u)
  C1 : Gain  Gain=sysest_ct.C  Multiplication=Matrix(K*u)
  Integrator2 : Integrator
  Sum7 : Sum  Inputs=|++
  system out : Outport
  states : Outport  Port=2
  wires:
  Sum7/1 -> Integrator2/1
  B1/1 -> Sum7/1
  Integrator2/1 -> states/1, A1/1, C1/1  "xhat"
  C1/1 -> system out/1  "y"
  A1/1 -> Sum7/2
  sat control signal/1 -> B1/1

== system Controllers_Complete_Comparisons/Plant3 ==
  sat control signal : Inport
  A1 : Gain  Gain=sysest_ct.A  Multiplication=Matrix(K*u)
  B1 : Gain  Gain=sysest_ct.B  Multiplication=Matrix(K*u)
  C1 : Gain  Gain=sysest_ct.C  Multiplication=Matrix(K*u)
  Integrator2 : Integrator
  Sum7 : Sum  Inputs=|++
  system out : Outport
  states : Outport  Port=2
  wires:
  Sum7/1 -> Integrator2/1
  B1/1 -> Sum7/1
  Integrator2/1 -> states/1, A1/1, C1/1  "xhat"
  C1/1 -> system out/1  "y"
  A1/1 -> Sum7/2
  sat control signal/1 -> B1/1

== system Controllers_Complete_Comparisons/Pole placement ==
  ref : Inport
  Xhat : Inport  Port=2
  Gain4 : Gain  Gain=K_p
  K : Gain  Gain=K_pp  Multiplication=Matrix(K*u)
  Sum1 : Sum  Inputs=|+-
  " control signal" : Outport
  wires:
  K/1 -> Sum1/2
  Xhat/1 -> K/1
  Sum1/1 -> " control signal"/1  "u"
  Gain4/1 -> Sum1/1
  ref/1 -> Gain4/1

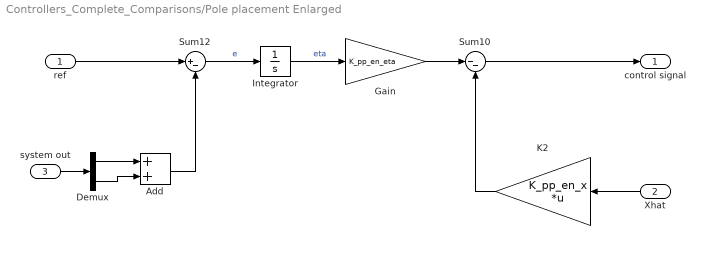
== system Controllers_Complete_Comparisons/Pole placement Enlarged ==
  ref : Inport
  Xhat : Inport  Port=2
  system out : Inport  Port=3
  Add : Sum
  Demux : Demux  Outputs=2
  Gain : Gain  Gain=K_pp_en_eta
  Integrator : Integrator
  K2 : Gain  Gain=K_pp_en_x  Multiplication=Matrix(K*u)
  Sum10 : Sum  Inputs=|--
  Sum12 : Sum  Inputs=|+-
  " control signal" : Outport
  wires:
  ref/1 -> Sum12/1
  Gain/1 -> Sum10/1
  Integrator/1 -> Gain/1  "eta"
  Sum10/1 -> " control signal"/1
  K2/1 -> Sum10/2
  Add/1 -> Sum12/2
  Sum12/1 -> Integrator/1  "e"
  Xhat/1 -> K2/1
  system out/1 -> Demux/1
  Demux/2 -> Add/2
  Demux/1 -> Add/1

== system Controllers_Complete_Comparisons/Pole placement PI ==
  ref : Inport
  Xhat : Inport  Port=2
  system out : Inport  Port=3
  Add : Sum
  Demux : Demux  Outputs=2
  K : Gain  Gain=K_pp  Multiplication=Matrix(K*u)
  LTI System1 : cstblocks/LTI System  sys=PI_pp  IC=[]
  Sum1 : Sum  Inputs=|+-
  Sum12 : Sum  Inputs=|+-
  " control signal" : Outport
  wires:
  K/1 -> Sum1/2
  Xhat/1 -> K/1
  Sum1/1 -> " control signal"/1  "u"
  LTI System1/1 -> Sum1/1
  Sum12/1 -> LTI System1/1  "e"
  Demux/1 -> Add/1
  system out/1 -> Demux/1
  Add/1 -> Sum12/2
  Demux/2 -> Add/2
  ref/1 -> Sum12/1

== system Controllers_Complete_Comparisons/Signal Builder1 ==
  Demux : Demux  Tag=STV Demux  Outputs=1
      settings: DisplayOption=none
  FromWs : FromWorkspace  Tag=STV FromWs  VariableName=tuvar
      SigBuilderData=|
      | common.afterFinalStr = 'Extrapolate'
      | common.sampleTime = 0
      | dataSet.timeRange = [0 10]
      | dataSet.name = 'Group 1'
      | sbobj.Groups.Name = 'Group 1'
      | sbobj.Groups.Signals.Name = 'Signal 1'
      | sbobj.Groups.Signals.XData = [0 1 1 3 3 5 5 7 7 8.5 8.5 10]
      | sbobj.Groups.Signals.YData = [0.005 0.005 40 40 15 15 -30 -30 0 0 23 23]
  Signal 1 : Outport  Tag=STV Outport
  wires:
  Demux/1 -> Signal 1/1
  FromWs/1 -> Demux/1

== system Controllers_Complete_Comparisons/State Extractor ==
  system out : Inport
  Demux7 : Demux  Outputs=2
  Derivative : Derivative
  Derivative1 : Derivative
  Mux2 : Mux
  Xhat : Outport
  wires:
  system out/1 -> Demux7/1
  Derivative1/1 -> Mux2/4  "alpha dot"
  Derivative/1 -> Mux2/2  "theta dot"
  Demux7/1 -> Mux2/1, Derivative/1  "theta"
  Demux7/2 -> Derivative1/1, Mux2/3  "alpha"
  Mux2/1 -> Xhat/1

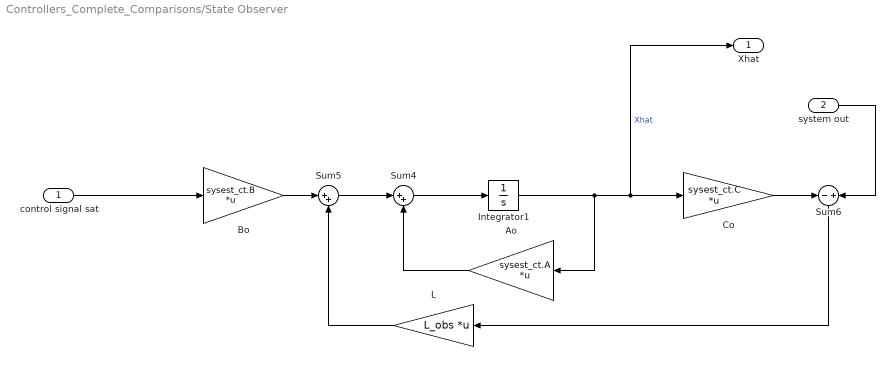
== system Controllers_Complete_Comparisons/State Observer ==
  control signal sat : Inport
  system out : Inport  Port=2
  Ao : Gain  Gain=sysest_ct.A  Multiplication=Matrix(K*u)
  Bo : Gain  Gain=sysest_ct.B  Multiplication=Matrix(K*u)
  Co : Gain  Gain=sysest_ct.C  Multiplication=Matrix(K*u)
  Integrator1 : Integrator
  L : Gain  Gain=L_obs  Multiplication=Matrix(K*u)
  Sum4 : Sum  Inputs=|++
  Sum5 : Sum  Inputs=|++
  Sum6 : Sum  Inputs=-+
  Xhat : Outport
  wires:
  system out/1 -> Sum6/2
  Ao/1 -> Sum4/2
  Sum4/1 -> Integrator1/1
  control signal sat/1 -> Bo/1
  Co/1 -> Sum6/1
  Sum6/1 -> L/1
  Bo/1 -> Sum5/1
  L/1 -> Sum5/2
  Integrator1/1 -> Xhat/1, Co/1, Ao/1  "Xhat"
  Sum5/1 -> Sum4/1

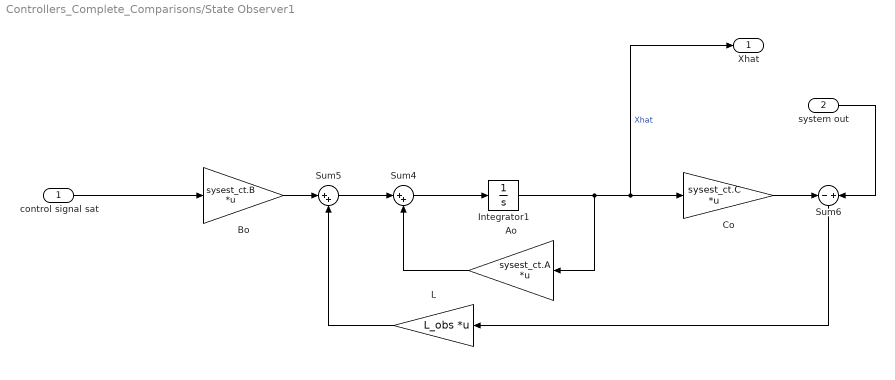
== system Controllers_Complete_Comparisons/State Observer1 ==
  control signal sat : Inport
  system out : Inport  Port=2
  Ao : Gain  Gain=sysest_ct.A  Multiplication=Matrix(K*u)
  Bo : Gain  Gain=sysest_ct.B  Multiplication=Matrix(K*u)
  Co : Gain  Gain=sysest_ct.C  Multiplication=Matrix(K*u)
  Integrator1 : Integrator
  L : Gain  Gain=L_obs  Multiplication=Matrix(K*u)
  Sum4 : Sum  Inputs=|++
  Sum5 : Sum  Inputs=|++
  Sum6 : Sum  Inputs=-+
  Xhat : Outport
  wires:
  system out/1 -> Sum6/2
  Ao/1 -> Sum4/2
  Sum4/1 -> Integrator1/1
  control signal sat/1 -> Bo/1
  Co/1 -> Sum6/1
  Sum6/1 -> L/1
  Bo/1 -> Sum5/1
  L/1 -> Sum5/2
  Integrator1/1 -> Xhat/1, Co/1, Ao/1  "Xhat"
  Sum5/1 -> Sum4/1

== system Controllers_Complete_Comparisons/State Observer2 ==
  control signal sat : Inport
  system out : Inport  Port=2
  Ao : Gain  Gain=sysest_ct.A  Multiplication=Matrix(K*u)
  Bo : Gain  Gain=sysest_ct.B  Multiplication=Matrix(K*u)
  Co : Gain  Gain=sysest_ct.C  Multiplication=Matrix(K*u)
  Integrator1 : Integrator
  L : Gain  Gain=L_obs  Multiplication=Matrix(K*u)
  Sum4 : Sum  Inputs=|++
  Sum5 : Sum  Inputs=|++
  Sum6 : Sum  Inputs=-+
  Xhat : Outport
  wires:
  system out/1 -> Sum6/2
  Ao/1 -> Sum4/2
  Sum4/1 -> Integrator1/1
  control signal sat/1 -> Bo/1
  Co/1 -> Sum6/1
  Sum6/1 -> L/1
  Bo/1 -> Sum5/1
  L/1 -> Sum5/2
  Integrator1/1 -> Xhat/1, Co/1, Ao/1  "Xhat"
  Sum5/1 -> Sum4/1

== system Controllers_Complete_Comparisons/State Observer3 ==
  control signal sat : Inport
  system out : Inport  Port=2
  Ao : Gain  Gain=sysest_ct.A  Multiplication=Matrix(K*u)
  Bo : Gain  Gain=sysest_ct.B  Multiplication=Matrix(K*u)
  Co : Gain  Gain=sysest_ct.C  Multiplication=Matrix(K*u)
  Integrator1 : Integrator
  L : Gain  Gain=L_obs  Multiplication=Matrix(K*u)
  Sum4 : Sum  Inputs=|++
  Sum5 : Sum  Inputs=|++
  Sum6 : Sum  Inputs=-+
  Xhat : Outport
  wires:
  system out/1 -> Sum6/2
  Ao/1 -> Sum4/2
  Sum4/1 -> Integrator1/1
  control signal sat/1 -> Bo/1
  Co/1 -> Sum6/1
  Sum6/1 -> L/1
  Bo/1 -> Sum5/1
  L/1 -> Sum5/2
  Integrator1/1 -> Xhat/1, Co/1, Ao/1  "Xhat"
  Sum5/1 -> Sum4/1

== system Controllers_Complete_Comparisons/State Observer4 ==
  control signal sat : Inport
  system out : Inport  Port=2
  Ao : Gain  Gain=sysest_ct.A  Multiplication=Matrix(K*u)
  Bo : Gain  Gain=sysest_ct.B  Multiplication=Matrix(K*u)
  Co : Gain  Gain=sysest_ct.C  Multiplication=Matrix(K*u)
  Integrator1 : Integrator
  L : Gain  Gain=L_obs  Multiplication=Matrix(K*u)
  Sum4 : Sum  Inputs=|++
  Sum5 : Sum  Inputs=|++
  Sum6 : Sum  Inputs=-+
  Xhat : Outport
  wires:
  system out/1 -> Sum6/2
  Ao/1 -> Sum4/2
  Sum4/1 -> Integrator1/1
  control signal sat/1 -> Bo/1
  Co/1 -> Sum6/1
  Sum6/1 -> L/1
  Bo/1 -> Sum5/1
  L/1 -> Sum5/2
  Integrator1/1 -> Xhat/1, Co/1, Ao/1  "Xhat"
  Sum5/1 -> Sum4/1

== matlab function Controllers_Complete_Comparisons/Kalman Filter Alp/MATLAB Function ==
  data: x_est input; y input; u input; x_est output; p_est input; p_est output; A input; B input; Q input; R input
function [x_est,p_est] = fcn(x_est,y,u,p_est, A,B,Q,R)
% Initialize state transition matrix
% Measurement matrix
H = [ 1 0 0 0; 0  0 1 0 ];


% Predicted state and covariance
x_prd = A * x_est + B* u;
p_prd = A * p_est * A' + Q;
% Estimation
S = p_prd'  + R;
B = p_prd';
klm_gain = (S \ B)';
% Estimated state and covariance
x_est = x_prd + klm_gain * (pinv(H)*y - x_prd);
p_est = p_prd - klm_gain  * p_prd;
% Compute the estimated measurements
end
